simulink library "Simple_House_ISOgm_CONF"  (R2016b)
settings: Solver=ode45  StartTime=0.0  StopTime=10.0  RelTol=1e-3  EnableMultiTasking=on
undefined symbols (not defined in the file): path_carnot
libraries: carnot x1
settings Model: Creator=lena.frank  LastModifiedBy=drhf
settings DataIOCC: LimitDataPoints=on  SaveFormat=Array  SignalLoggingSaveFormat=ModelDataLogs
settings OptimizationCC: ExpressionDepthLimit=2147483647  LifeSpan=inf
settings DebuggingCC: UnderspecifiedInitializationDetection=Classic  MergeDetectMultiDrivingBlocksExec=none  SolverPrmCheckMsg=warning  FcnCallInpInsideContextMsg=warning  StateNameClashWarn=warning  SFUnexpectedBacktrackingDiag=warning  SFNoUnconditionalDefaultTransitionDiag=warning  SFExecutionAtInitializationDiag=none
settings HardwareCC: ProdBitPerPointer=32  ProdBitPerSizeT=32  ProdBitPerPtrDiffT=32  ProdLargestAtomicFloat=None  ProdIntDivRoundTo=Undefined  ProdEndianess=Unspecified  ProdWordSize=32  ProdHWDeviceType=32-bit Generic
settings ModelReferenceCC: PropagateSignalLabelsOutOfModel=off
settings GRTTargetCC: TargetLangStandard=C89/C90 (ANSI)  GeneratePreprocessorConditionals=Disable all  CombineOutputUpdateFcns=off  GRTInterface=on
settings ConfigComp: CovMetricSettings=dw  CovHtmlReporting=on  CovSaveCumulativeToWorkspaceVar=on  CovSaveSingleToWorkspaceVar=on  CovExternalEMLEnable=off

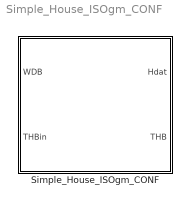
== system Simple_House_ISOgm_CONF ==
  Simple_House_ISOgm_CONF : Subsystem  mask(Simple House with ISO 13370 Ground Model){tini=20, PathName=fullfile(path_carnot('libsl'),'Load','Houses','Simple_House_ISOgm_CONF','parameter_set'), FileName='Default_SimpleHouseISOgm.mat', userPath=off, userParam=off, Ahabit=140, Hroom=2.5, Slab=[7 10], UAwall=100, UAneighbour=0, Uground=0.7, cap=70000000, Awindow=[12 4 3 4], AziWindow=[0 90 -180 -90], Uwindow=[2 2 2 2], Gwindow=[0.5 0.5 0.5 0.5], shading=0.75, Ventilationrate=0.4, Heatrecovery=0, Heatload=4500, DTnomHeatingsystem=15, RadiatorExponent=1.1, CapHeatingsystem=40000000, DpHeatingsystem=[10 10]}
      mask prompts: tini "Initial temperature in °C"; PathName "Path"; FileName "Parameter set"; userPath "Edit path and name of parameter set"; userParam "User defined parameters"; Ahabit "Living surface in m²"; Hroom "height of rooms in m"; Slab "Dimensions of slab in m [length width]"; UAwall "Total heat transfer to ambient (walls/roof) in W/K"; UAneighbour "Total heat transfer to neighbour inW/K"; Uground "Heat transfer coeffient of slab to ground in W/m²/K"; cap "Total thermal capacity in J/K"; Awindow "Surface of 4 windows in m² (vector)"; AziWindow "Orientation of 4 windows (south 0, east -90,west 90)"; Uwindow "Heat loss coefficient 4 windows in W/m²/K [vector]"; Gwindow "Light transmittance 4 windows (0..1) * (1 - frame_part) [vector]"; shading "Shading factor [0..1] when T room > 4 K + T_init"; Ventilationrate "Ventilation rate in 1/h"; Heatrecovery "Heat recovery (0..1)"; Heatload "Heating capacity radiator  [W]"; DTnomHeatingsystem "Nominal delta T (average radiator temperature - room temperature) [K]"; RadiatorExponent "Radiator exponent"; CapHeatingsystem "Mass*capacity of heating system [J/K]"; DpHeatingsystem "Pressure drop coefficients [linear quadratic] in Pa/(kg/s), Pa/(kg/s)²"
      mask help:
      | Configurated building model, variables are defined in a mat-file (for example in "Default_SimpleHouseISOgm.mat") in the folder /parameter_set of the block.
      | Use of buttons in the "Picking a file" frame:
      | 1) "Carnot public data" choses a parameter file from the public data folder in Carnot. The "Path" is set to the public data folder.
      | 2) "Carnot internal data" choses a parameter file from the internal data folder in Carnot. The "Path" is set to the internal data folder.
      | 3) "From selected path" choses a parameter file from the "Path".
      | Allow editing "File" and "Path" with the checkbox. Be aware that the buttons in the "Picking a file" frame will anyway overwrite the edited values.
      mask init:
      | [ok, param] = CarnotCallbacks_SimpleHouseISOgmConf('SetParameters',gcbh,PathName,FileName);
      mask Help: web(fullfile(path_carnot('help'),'simple_house.html'),'-helpbrowser')
      mask TypeOptions tini: Simple_House_ISO_GroundModel/tini
      mask Callback userPath: [ok, param] = CarnotCallbacks_SimpleHouseISOgmConf('UserEdit',gcbh);
      mask Callback userParam: [ok, param] = CarnotCallbacks_SimpleHouseISOgmConf('UserEdit',gcbh);
      mask TypeOptions Ahabit: Simple_House_ISO_GroundModel/Ahabit
      mask TypeOptions Hroom: Simple_House_ISO_GroundModel/Hroom
      mask TypeOptions Slab: Simple_House_ISO_GroundModel/Floorsize
      mask TypeOptions UAwall: Simple_House_ISO_GroundModel/UAwall
      mask TypeOptions UAneighbour: Simple_House_ISO_GroundModel/UAneighbour
      mask TypeOptions Uground: Simple_House_ISO_GroundModel/Uground
      mask TypeOptions cap: Simple_House_ISO_GroundModel/mc
      mask TypeOptions Awindow: Simple_House_ISO_GroundModel/Awin
      mask TypeOptions AziWindow: Simple_House_ISO_GroundModel/AziWin
      mask TypeOptions Uwindow: Simple_House_ISO_GroundModel/Uwin
      mask TypeOptions Gwindow: Simple_House_ISO_GroundModel/Gwin
      mask TypeOptions shading: Simple_House_ISO_GroundModel/shade
      mask TypeOptions Ventilationrate: Simple_House_ISO_GroundModel/vent
      mask TypeOptions Heatrecovery: Simple_House_ISO_GroundModel/rec
      mask TypeOptions Heatload: Simple_House_ISO_GroundModel/heatload
      mask TypeOptions DTnomHeatingsystem: Simple_House_ISO_GroundModel/delta_t_nom
      mask TypeOptions RadiatorExponent: Simple_House_ISO_GroundModel/n_rad
      mask TypeOptions CapHeatingsystem: Simple_House_ISO_GroundModel/mass_times_cap
      mask TypeOptions DpHeatingsystem: Simple_House_ISO_GroundModel/dpcoeff
      mask DialogControl Control1 Prompt: Carnot public data
      mask DialogControl Control1 Callback: [ok, file] = CarnotCallbacks_SimpleHouseISOgmConf('GetFilename',gcbh, 'public');
      mask DialogControl Control3 Prompt: Carnot internal data
      mask DialogControl Control3 Callback: [ok, file] = CarnotCallbacks_SimpleHouseISOgmConf('GetFilename',gcbh, 'internal');
      mask DialogControl Control4 Prompt: Selected path
      mask DialogControl Control4 Callback: [ok, file] = CarnotCallbacks_SimpleHouseISOgmConf('GetFilename',gcbh, 'selected');
      mask DialogControl Control5 Prompt: Save in Carnot internal data
      mask DialogControl Control5 Callback: [ok, param] = CarnotCallbacks_SimpleHouseISOgmConf('SaveFilename',gcbh, 'internal','SH');
      mask DialogControl Control6 Prompt: Save in selected path
      mask DialogControl Control6 Callback: [ok, param] = CarnotCallbacks_SimpleHouseISOgmConf('SaveFilename',gcbh, 'selected','SH');
      mask Display:
      | % user defined picture file
      | picfile = fullfile(path_carnot('intlibsl'), ...
      |         'Load','Houses','Simple_House_ISOgm_CONF','parameter_set', ...
      |         'Simple_House_ISOgm_CONF.jpg');
      | 
      | % show internal picture if defined
      | if ~BlockIsInCarnotLibrary ...      % if not located in library any more
      |         && exist(picfile,'file')    % AND picfile is present
      |     image(imread(picfile), [0.15 0.1 0.7 0.8])
      |     set_param(gcb, 'BackgroundColor', 'White')
      | else
      |     % show public picture
      |     plot([10,10,90,90,10]/100,[0,50,50,0,0]/100,...
      |          [100,60,40,0]/100,[40,80,80,40]/100,...
      |          [20,34,34,20,20]/100,[40,40,20,20,40]/100,...
      |          [60,60,40,40]/100,[0,40,40,0]/100,...
      |          [65,80,80,65,65]/100,[40,40,20,20,40]/100,...
      |          [47,54,54,47,47]/100,[35,35,4,4,35]/100,...
      |          [45,41]/100,[20,20]/100)
      |     set_param(gcb, 'BackgroundColor', 'Orange')
      | end
      | 
      | % port labels
      | % port_label('input',1,'WDB')
      | % port_label('input',2,'THB')
      | % port_label('output',1,'Hdat')
      | % port_label('output',2,'THB')

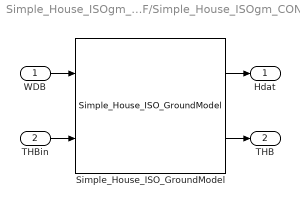
== system Simple_House_ISOgm_CONF/Simple_House_ISOgm_CONF ==
  WDB : Inport
  THBin : Inport  Port=2
  Simple_House_ISO_GroundModel : carnot/Load/Houses/Simple_House_ISO_GroundModel  Ahabit=Ahabit  Hroom=Hroom  Floorsize=Slab  UAwall=UAwall  UAneighbour=UAneighbour  Uground=Uground  mc=cap  shade=shading  tini=tini  Awin=Awindow  AziWin=AziWindow  Uwin=Uwindow  Gwin=Gwindow  vent=Ventilationrate  rec=Heatrecovery  heatload=Heatload  delta_t_nom=DTnomHeatingsystem  n_rad=RadiatorExponent  mass_times_cap=CapHeatingsystem  dpcoeff=DpHeatingsystem
  Hdat : Outport
  THB : Outport  Port=2
  wires:
  WDB/1 -> Simple_House_ISO_GroundModel/1
  Simple_House_ISO_GroundModel/1 -> Hdat/1
  THBin/1 -> Simple_House_ISO_GroundModel/2
  Simple_House_ISO_GroundModel/2 -> THB/1
